simulink model "VehicleModelBusTest"  (R2020b)
settings: Solver=VariableStepAuto  StartTime=0.0  StopTime=10.0  RelTol=1e-3
settings Model: Creator=Authorized User  LastModifiedBy=Authorized User

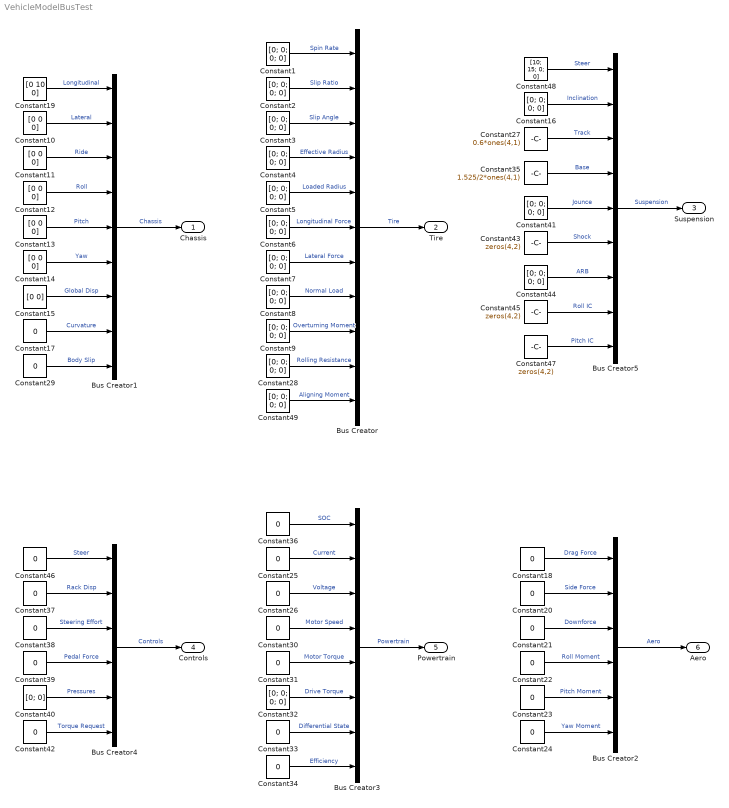
== system VehicleModelBusTest ==
  Bus Creator : BusCreator  Inputs=11
  Bus Creator1 : BusCreator  Inputs=9
  Bus Creator2 : BusCreator  Inputs=6
  Bus Creator3 : BusCreator  Inputs=8
  Bus Creator4 : BusCreator  Inputs=6
  Bus Creator5 : BusCreator  Inputs=9
  Constant{1..9,16,28,32,41,44,49} (15 alike) : Constant  Value=[0; 0; 0; 0]
  Constant{10..14} (5 alike) : Constant  Value=[0 0 0]
  Constant15 : Constant  Value=[0 0]
  Constant{17..18,20..26,29..31,33..34,36..39,42,46} (20 alike) : Constant  Value=0
  Constant19 : Constant  Value=[0 10 0]
  Constant27 : Constant  Value=0.6*ones(4,1)
  Constant35 : Constant  Value=1.525/2*ones(4,1)
  Constant40 : Constant  Value=[0; 0]
  Constant43 : Constant  Value=zeros(4,2)
  Constant45 : Constant  Value=zeros(4,2)
  Constant47 : Constant  Value=zeros(4,2)
  Constant48 : Constant  Value=[10; 15; 0; 0]
  Chassis : Outport  OutDataTypeStr=Bus: Chassis
  Tire : Outport  Port=2  OutDataTypeStr=Bus: Tire
  Suspension : Outport  Port=3  OutDataTypeStr=Bus: Suspension
  Controls : Outport  Port=4  OutDataTypeStr=Bus: Controls
  Powertrain : Outport  Port=5  OutDataTypeStr=Bus: Powertrain
  Aero : Outport  Port=6  OutDataTypeStr=Bus: Aero
  wires:
  Constant2/1 -> Bus Creator/2  "Slip Ratio"
  Constant3/1 -> Bus Creator/3  "Slip Angle"
  Constant4/1 -> Bus Creator/4  "Effective Radius"
  Constant6/1 -> Bus Creator/6  "Longitudinal Force"
  Constant7/1 -> Bus Creator/7  "Lateral Force"
  Constant8/1 -> Bus Creator/8  "Normal Load"
  Constant9/1 -> Bus Creator/9  "Overturning Moment"
  Constant28/1 -> Bus Creator/10  "Rolling Resistance"
  Constant49/1 -> Bus Creator/11  "Aligning Moment"
  Constant1/1 -> Bus Creator/1  "Spin Rate"
  Bus Creator/1 -> Tire/1  "Tire"
  Bus Creator1/1 -> Chassis/1  "Chassis"
  Constant11/1 -> Bus Creator1/3  "Ride"
  Constant12/1 -> Bus Creator1/4  "Roll"
  Constant14/1 -> Bus Creator1/6  "Yaw"
  Constant10/1 -> Bus Creator1/2  "Lateral"
  Constant19/1 -> Bus Creator1/1  "Longitudinal"
  Constant13/1 -> Bus Creator1/5  "Pitch"
  Constant15/1 -> Bus Creator1/7  "Global Disp"
  Bus Creator2/1 -> Aero/1  "Aero"
  Constant18/1 -> Bus Creator2/1  "Drag Force"
  Constant20/1 -> Bus Creator2/2  "Side Force"
  Constant21/1 -> Bus Creator2/3  "Downforce"
  Constant22/1 -> Bus Creator2/4  "Roll Moment"
  Constant23/1 -> Bus Creator2/5  "Pitch Moment"
  Constant24/1 -> Bus Creator2/6  "Yaw Moment"
  Bus Creator3/1 -> Powertrain/1  "Powertrain"
  Constant26/1 -> Bus Creator3/3  "Voltage"
  Constant33/1 -> Bus Creator3/7  "Differential State"
  Constant31/1 -> Bus Creator3/5  "Motor Torque"
  Constant25/1 -> Bus Creator3/2  "Current"
  Constant36/1 -> Bus Creator3/1  "SOC"
  Constant34/1 -> Bus Creator3/8  "Efficiency"
  Constant30/1 -> Bus Creator3/4  "Motor Speed"
  Constant32/1 -> Bus Creator3/6  "Drive Torque"
  Constant38/1 -> Bus Creator4/3  "Steering Effort"
  Bus Creator4/1 -> Controls/1  "Controls"
  Constant40/1 -> Bus Creator4/5  "Pressures"
  Constant46/1 -> Bus Creator4/1  "Steer"
  Constant37/1 -> Bus Creator4/2  "Rack Disp"
  Constant39/1 -> Bus Creator4/4  "Pedal Force"
  Constant17/1 -> Bus Creator1/8  "Curvature"
  Constant29/1 -> Bus Creator1/9  "Body Slip"
  Constant42/1 -> Bus Creator4/6  "Torque Request"
  Constant27/1 -> Bus Creator5/3  "Track"
  Bus Creator5/1 -> Suspension/1  "Suspension"
  Constant41/1 -> Bus Creator5/5  "Jounce"
  Constant44/1 -> Bus Creator5/7  "ARB"
  Constant48/1 -> Bus Creator5/1  "Steer"
  Constant16/1 -> Bus Creator5/2  "Inclination"
  Constant35/1 -> Bus Creator5/4  "Base"
  Constant43/1 -> Bus Creator5/6  "Shock"
  Constant47/1 -> Bus Creator5/9  "Pitch IC"
  Constant45/1 -> Bus Creator5/8  "Roll IC"
  Constant5/1 -> Bus Creator/5  "Loaded Radius"
